simulink model "linearization"  (R2023b)
settings: Solver=ode3  StartTime=0.0  StopTime=20  FixedStep=0.01  RelTol=1e-3  EnableMultiTasking=on
undefined symbols (not defined in the file or in its folder): dNx, dNy, dSx, dSy, g, kFD, kFT_N, kFT_S, kMD, kMDR_N, kMDR_S, m, w_hov
libraries: shared6dof x1
settings Model: Creator=rcasado  LastModifiedBy=Rafa
settings SolverCC: AlgebraicLoopSolver=TrustRegion
settings DataIOCC: LimitDataPoints=on  SaveFormat=Array  ReturnWorkspaceOutputs=off
settings OptimizationCC: ReuseModelBlockBuffer=off  LifeSpan=inf
settings DebuggingCC: MultiTaskRateTransMsg=warning  UnconnectedInputMsg=warning  UnconnectedOutputMsg=warning  UnconnectedLineMsg=warning  AllowSymbolicDim=off  SFUnexpectedBacktrackingDiag=warning  SFNoUnconditionalDefaultTransitionDiag=warning  SFExecutionAtInitializationDiag=none  ArithmeticOperatorsInVariantConditions=warning
settings HardwareCC: ProdBitPerPointer=32  ProdBitPerSizeT=32  ProdBitPerPtrDiffT=32  ProdLargestAtomicFloat=None  ProdIntDivRoundTo=Undefined  ProdEndianess=Unspecified  ProdWordSize=32  ProdHWDeviceType=32-bit Generic
settings ModelReferenceCC: EnableRefExpFcnMdlSchedulingChecks=on  PropagateSignalLabelsOutOfModel=off
settings SFSimCC: SimUseLocalCustomCode=off  CustomCodeUndefinedFunction=UseInterfaceOnly
settings RTWCC: RTWUseLocalCustomCode=off
settings CodeAppCC: StateflowObjectComments=on
settings GRTTargetCC: TargetLangStandard=C89/C90 (ANSI)
settings ConfigComp: CovMetricSettings=dw  CovSaveCumulativeToWorkspaceVar=on  CovSaveSingleToWorkspaceVar=on  CovExternalEMLEnable=off

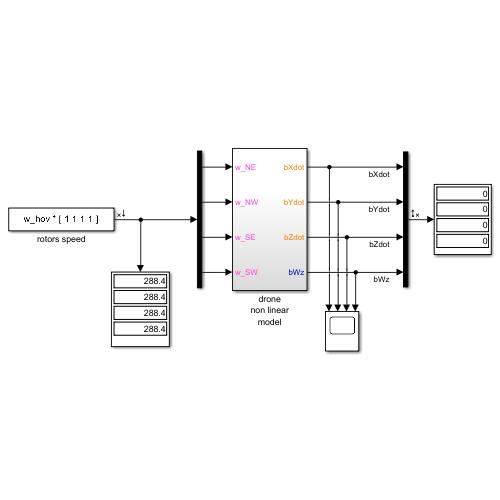
[thumbnail: Simulink's stored preview of the top-level diagram]
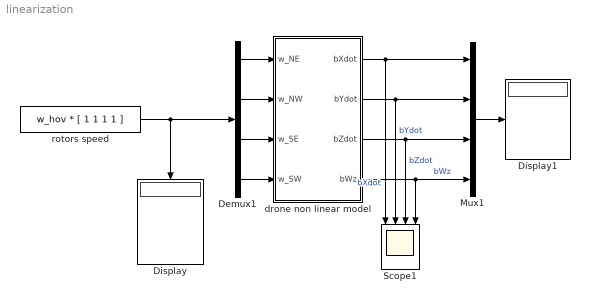
== system linearization ==
  Demux1 : Demux
  Display : Display
  Display1 : Display
  Mux1 : Mux
  Scope1 : Scope  NumInputPorts=4
  drone non linear model : Subsystem
  rotors speed : Constant  Value=w_hov * [ 1 1 1 1 ]
  wires:
  Demux1/3 -> drone non linear model/3(w_SE)
  Demux1/2 -> drone non linear model/2(w_NW)
  Mux1/1 -> Display1/1
  rotors speed/1 -> Demux1/1, Display/1
  drone non linear model/1(bXdot) -> Mux1/1, Scope1/1  "bXdot"
  drone non linear model/3(bZdot) -> Mux1/3, Scope1/3  "bZdot"
  drone non linear model/2(bYdot) -> Mux1/2, Scope1/2  "bYdot"
  Demux1/4 -> drone non linear model/4(w_SW)
  Demux1/1 -> drone non linear model/1(w_NE)
  drone non linear model/4(bWz) -> Mux1/4, Scope1/4  "bWz"

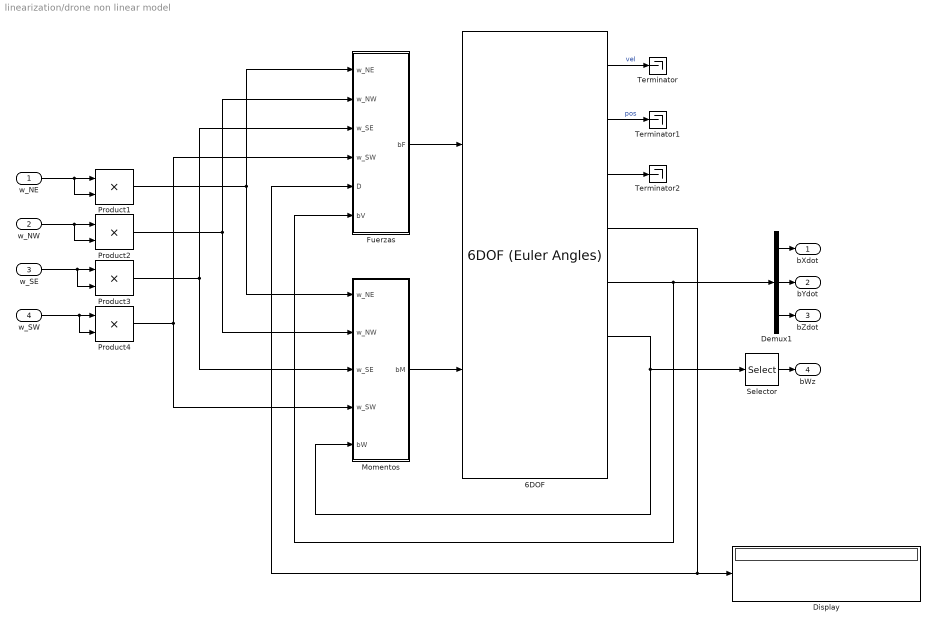
== system linearization/drone non linear model ==
  w_NE : Inport
  w_NW : Inport  Port=2
  w_SE : Inport  Port=3
  w_SW : Inport  Port=4
  6DOF : shared6dof/6DOF (Euler Angles)  units=Metric (MKS)  mtype=Fixed  rep=Euler Angles  xme_0=[0 0 0]  Vm_0=[0 0 0]  eul_0=[0 0 0]  pm_0=[0 0 0]  mass_0=m  mass_e=0.5  mass_f=2.0  inertia=inertia  inertia_e=eye(3)  inertia_f=2*eye(3)  k_quat=1.0  vre_flag=on  abi_flag=off  aMode=aMode  xme_statename=''  Vm_statename=''  eul_statename=''  quat_statename=''  pm_statename=''  mass_statename=''
  Demux1 : Demux  Outputs=3
  Display : Display
  Fuerzas : Subsystem
  Momentos : Subsystem
  Product{1..4} (4 alike) : Product
  Selector : Selector  InputPortWidth=3  IndexOptions=Index vector (dialog)  Indices=[3]  OutputSizes=1
  Terminator : Terminator
  Terminator1 : Terminator
  Terminator2 : Terminator
  bXdot : Outport  VectorParamsAs1DForOutWhenUnconnected=off
  bYdot : Outport  Port=2  VectorParamsAs1DForOutWhenUnconnected=off
  bZdot : Outport  Port=3  VectorParamsAs1DForOutWhenUnconnected=off
  bWz : Outport  Port=4  VectorParamsAs1DForOutWhenUnconnected=off
  wires:
  Momentos/1(bM) -> 6DOF/2
  6DOF/4 -> Fuerzas/5(D), Display/1
  Fuerzas/1(bF) -> 6DOF/1
  6DOF/6 -> Momentos/5(bW), Selector/1
  6DOF/5 -> Fuerzas/6(bV), Demux1/1
  Demux1/1 -> bXdot/1
  Demux1/2 -> bYdot/1
  Demux1/3 -> bZdot/1
  Selector/1 -> bWz/1
  6DOF/1 -> Terminator/1  "vel"
  6DOF/2 -> Terminator1/1  "pos"
  6DOF/3 -> Terminator2/1
  w_SW/1 -> Product4/2, Product4/1
  w_SE/1 -> Product3/2, Product3/1
  w_NW/1 -> Product2/2, Product2/1
  w_NE/1 -> Product1/2, Product1/1
  Product1/1 -> Fuerzas/1(w_NE), Momentos/1(w_NE)
  Product2/1 -> Fuerzas/2(w_NW), Momentos/2(w_NW)
  Product3/1 -> Fuerzas/3(w_SE), Momentos/3(w_SE)
  Product4/1 -> Fuerzas/4(w_SW), Momentos/4(w_SW)

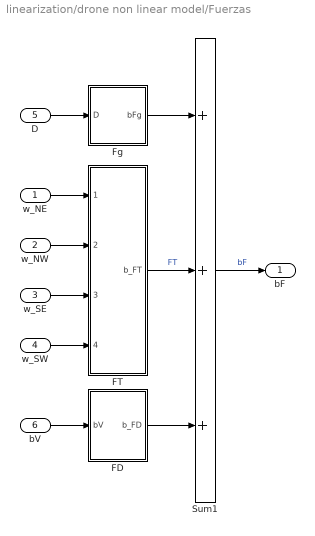
== system linearization/drone non linear model/Fuerzas ==
  w_NE : Inport
  w_NW : Inport  Port=2
  w_SE : Inport  Port=3
  w_SW : Inport  Port=4
  D : Inport  Port=5
  bV : Inport  Port=6
  FD : Subsystem
  FT : Subsystem
  Fg : Subsystem
  Sum1 : Sum  Inputs=+++
  bF : Outport  VectorParamsAs1DForOutWhenUnconnected=off
  wires:
  D/1 -> Fg/1(D)
  Fg/1(bFg) -> Sum1/1
  FT/1(b_FT) -> Sum1/2  "FT"
  w_SW/1 -> FT/4(w_SW)
  w_NE/1 -> FT/1(w_NE)
  w_SE/1 -> FT/3(w_SE)
  w_NW/1 -> FT/2(w_NW)
  Sum1/1 -> bF/1  "bF"
  bV/1 -> FD/1(bV)
  FD/1(b_FD) -> Sum1/3

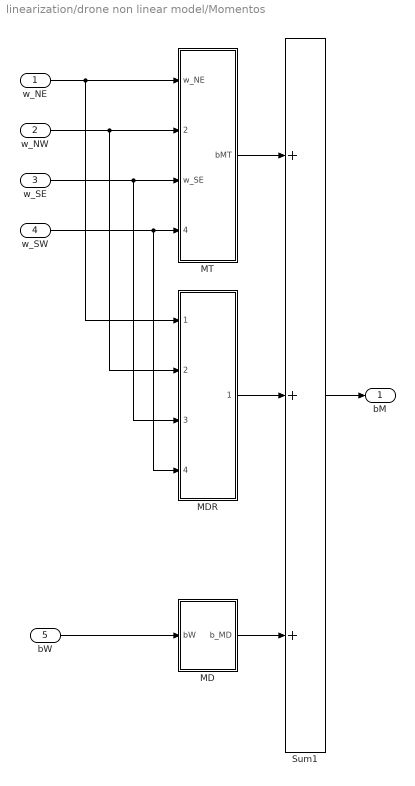
== system linearization/drone non linear model/Momentos ==
  w_NE : Inport
  w_NW : Inport  Port=2
  w_SE : Inport  Port=3
  w_SW : Inport  Port=4
  bW : Inport  Port=5
  MD : Subsystem
  MDR : Subsystem
  MT : Subsystem
  Sum1 : Sum  Inputs=+++
  bM : Outport  VectorParamsAs1DForOutWhenUnconnected=off
  wires:
  bW/1 -> MD/1(bW)
  MT/1(bMT) -> Sum1/1
  w_SW/1 -> MDR/4(w_SW), MT/4(w_SW)
  w_NE/1 -> MDR/1(w_NE), MT/1(w_NE)
  w_SE/1 -> MDR/3(w_SE), MT/3(w_SE)
  w_NW/1 -> MDR/2(w_NW), MT/2(w_NW)
  Sum1/1 -> bM/1
  MD/1(b_MD) -> Sum1/3
  MDR/1(b_MDR) -> Sum1/2

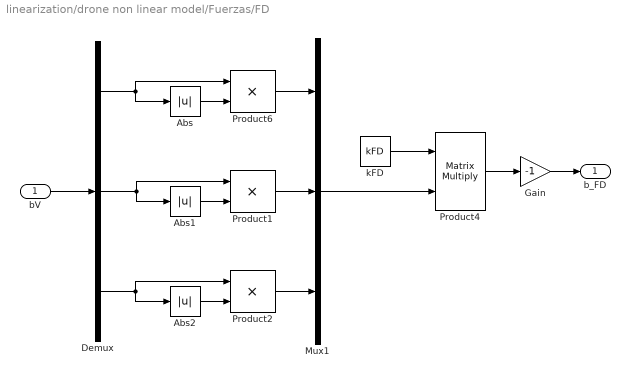
== system linearization/drone non linear model/Fuerzas/FD ==
  bV : Inport
  Abs : Abs  SaturateOnIntegerOverflow=off
  Abs1 : Abs  SaturateOnIntegerOverflow=off
  Abs2 : Abs  SaturateOnIntegerOverflow=off
  Demux : Demux  Outputs=3
  Gain : Gain  Gain=-1
  Mux1 : Mux  Inputs=3
  Product1 : Product
  Product2 : Product
  Product4 : Product  Multiplication=Matrix(*)
  Product6 : Product
  kFD : Constant  Value=kFD
  b_FD : Outport  VectorParamsAs1DForOutWhenUnconnected=off
  wires:
  kFD/1 -> Product4/1
  Product4/1 -> Gain/1
  Mux1/1 -> Product4/2
  Product1/1 -> Mux1/2
  bV/1 -> Demux/1
  Abs/1 -> Product6/2
  Abs1/1 -> Product1/2
  Abs2/1 -> Product2/2
  Demux/1 -> Product6/1, Abs/1
  Demux/2 -> Product1/1, Abs1/1
  Demux/3 -> Product2/1, Abs2/1
  Product6/1 -> Mux1/1
  Product2/1 -> Mux1/3
  Gain/1 -> b_FD/1

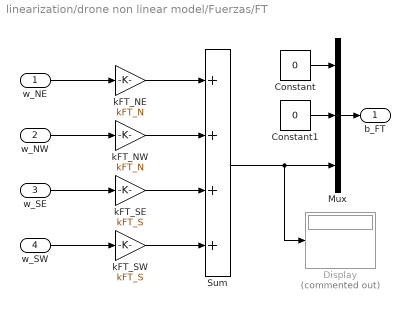
== system linearization/drone non linear model/Fuerzas/FT ==
  w_NE : Inport
  w_NW : Inport  Port=2
  w_SE : Inport  Port=3
  w_SW : Inport  Port=4
  Constant : Constant  Value=0
  Constant1 : Constant  Value=0
  Display : Display  Commented=on
  Mux : Mux  Inputs=3
  Sum : Sum  Inputs=++++
  kFT_NE : Gain  Gain=kFT_N
  kFT_NW : Gain  Gain=kFT_N
  kFT_SE : Gain  Gain=kFT_S
  kFT_SW : Gain  Gain=kFT_S
  b_FT : Outport  VectorParamsAs1DForOutWhenUnconnected=off
  wires:
  Mux/1 -> b_FT/1
  Constant/1 -> Mux/1
  Constant1/1 -> Mux/2
  Sum/1 -> Display/1, Mux/3
  w_NE/1 -> kFT_NE/1
  w_NW/1 -> kFT_NW/1
  w_SE/1 -> kFT_SE/1
  w_SW/1 -> kFT_SW/1
  kFT_NW/1 -> Sum/2
  kFT_NE/1 -> Sum/1
  kFT_SW/1 -> Sum/4
  kFT_SE/1 -> Sum/3

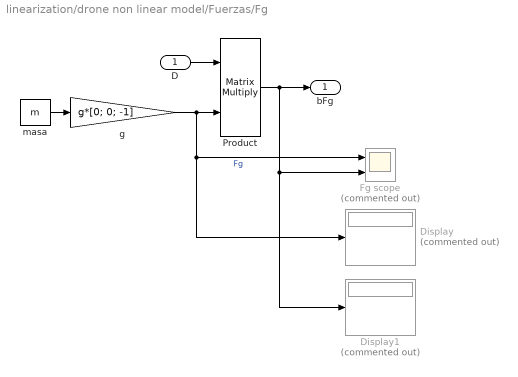
== system linearization/drone non linear model/Fuerzas/Fg ==
  D : Inport
  Display : Display  Commented=on
  Display1 : Display  Commented=on
  Fg scope : Scope  Commented=on  NumInputPorts=2
  Product : Product  Multiplication=Matrix(*)
  g : Gain  Gain=g*[0; 0; -1]
  masa : Constant  Value=m
  bFg : Outport  VectorParamsAs1DForOutWhenUnconnected=off
  wires:
  Product/1 -> Display1/1, Fg scope/2, bFg/1
  D/1 -> Product/1
  masa/1 -> g/1
  g/1 -> Display/1, Fg scope/1, Product/2  "Fg"

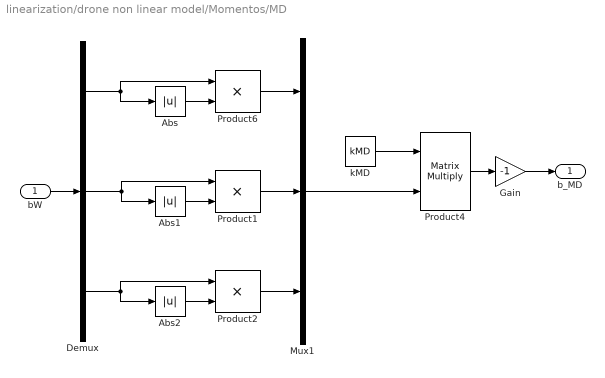
== system linearization/drone non linear model/Momentos/MD ==
  bW : Inport
  Abs : Abs  SaturateOnIntegerOverflow=off
  Abs1 : Abs  SaturateOnIntegerOverflow=off
  Abs2 : Abs  SaturateOnIntegerOverflow=off
  Demux : Demux  Outputs=3
  Gain : Gain  Gain=-1
  Mux1 : Mux  Inputs=3
  Product1 : Product
  Product2 : Product
  Product4 : Product  Multiplication=Matrix(*)
  Product6 : Product
  kMD : Constant  Value=kMD
  b_MD : Outport  VectorParamsAs1DForOutWhenUnconnected=off
  wires:
  kMD/1 -> Product4/1
  Product4/1 -> Gain/1
  Mux1/1 -> Product4/2
  Product1/1 -> Mux1/2
  bW/1 -> Demux/1
  Abs/1 -> Product6/2
  Abs1/1 -> Product1/2
  Abs2/1 -> Product2/2
  Demux/1 -> Product6/1, Abs/1
  Demux/2 -> Product1/1, Abs1/1
  Demux/3 -> Product2/1, Abs2/1
  Product6/1 -> Mux1/1
  Product2/1 -> Mux1/3
  Gain/1 -> b_MD/1

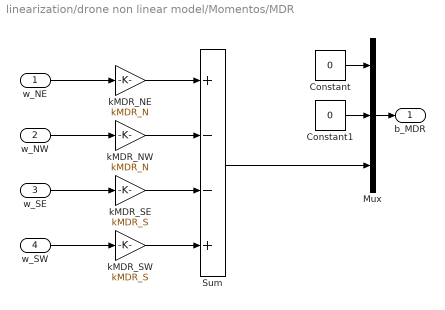
== system linearization/drone non linear model/Momentos/MDR ==
  w_NE : Inport
  w_NW : Inport  Port=2
  w_SE : Inport  Port=3
  w_SW : Inport  Port=4
  Constant : Constant  Value=0
  Constant1 : Constant  Value=0
  Mux : Mux  Inputs=3
  Sum : Sum  Inputs=+--+
  kMDR_NE : Gain  Gain=kMDR_N
  kMDR_NW : Gain  Gain=kMDR_N
  kMDR_SE : Gain  Gain=kMDR_S
  kMDR_SW : Gain  Gain=kMDR_S
  b_MDR : Outport  VectorParamsAs1DForOutWhenUnconnected=off
  wires:
  kMDR_SW/1 -> Sum/4
  kMDR_SE/1 -> Sum/3
  kMDR_NW/1 -> Sum/2
  kMDR_NE/1 -> Sum/1
  Mux/1 -> b_MDR/1
  Constant/1 -> Mux/1
  Constant1/1 -> Mux/2
  Sum/1 -> Mux/3
  w_SW/1 -> kMDR_SW/1
  w_SE/1 -> kMDR_SE/1
  w_NE/1 -> kMDR_NE/1
  w_NW/1 -> kMDR_NW/1

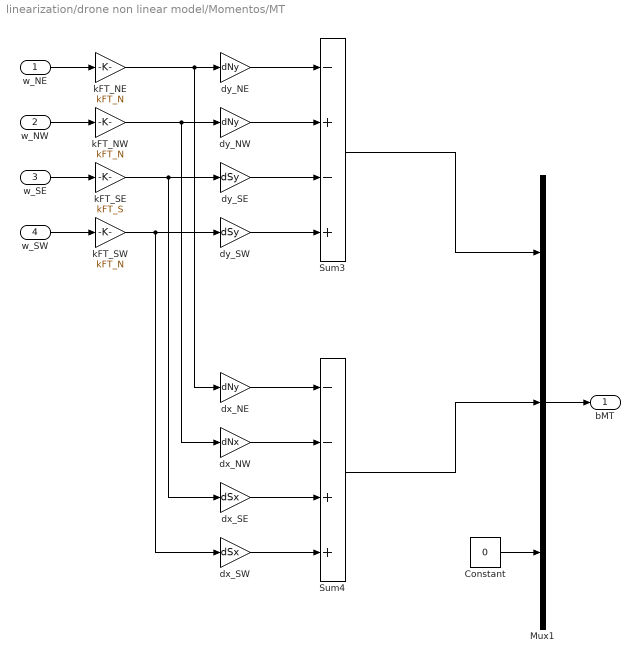
== system linearization/drone non linear model/Momentos/MT ==
  w_NE : Inport
  w_NW : Inport  Port=2
  w_SE : Inport  Port=3
  w_SW : Inport  Port=4
  Constant : Constant  Value=0
  Mux1 : Mux  Inputs=3
  Sum3 : Sum  Inputs=-+-+
  Sum4 : Sum  Inputs=--++
  dx_NE : Gain  Gain=dNy
  dx_NW : Gain  Gain=dNx
  dx_SE : Gain  Gain=dSx
  dx_SW : Gain  Gain=dSx
  dy_NE : Gain  Gain=dNy
  dy_NW : Gain  Gain=dNy
  dy_SE : Gain  Gain=dSy
  dy_SW : Gain  Gain=dSy
  kFT_NE : Gain  Gain=kFT_N
  kFT_NW : Gain  Gain=kFT_N
  kFT_SE : Gain  Gain=kFT_S
  kFT_SW : Gain  Gain=kFT_N
  bMT : Outport  VectorParamsAs1DForOutWhenUnconnected=off
  wires:
  Mux1/1 -> bMT/1
  Constant/1 -> Mux1/3
  kFT_NW/1 -> dx_NW/1, dy_NW/1
  kFT_NE/1 -> dx_NE/1, dy_NE/1
  kFT_SW/1 -> dx_SW/1, dy_SW/1
  w_NE/1 -> kFT_NE/1
  w_SE/1 -> kFT_SE/1
  kFT_SE/1 -> dx_SE/1, dy_SE/1
  w_NW/1 -> kFT_NW/1
  w_SW/1 -> kFT_SW/1
  dy_SE/1 -> Sum3/3
  dy_SW/1 -> Sum3/4
  dy_NE/1 -> Sum3/1
  dy_NW/1 -> Sum3/2
  dx_NW/1 -> Sum4/2
  dx_NE/1 -> Sum4/1
  dx_SW/1 -> Sum4/4
  dx_SE/1 -> Sum4/3
  Sum3/1 -> Mux1/1
  Sum4/1 -> Mux1/2
